simulink model "GHAME_Model_2018b"  (R2018b)
settings: Solver=ode2  StartTime=0.0  StopTime=Sim.simulation.duration  FixedStep=Sim.sample_time  RelTol=1e-3
undefined symbols (not defined in the file): Data, IC, Sim, UNC, v0_BE_B
libraries: simulink_extras x8, sharedutil x2
(part 1 of 2)
settings Model: PauseTimes=399.98  EnablePacing=on  PacingRate=5  Creator=Thoma  LastModifiedBy=muel_td
settings SolverCC: PositivePriorityOrder=on  MinimalZcImpactIntegration=on
settings DataIOCC: ExternalInput=getinputstruct(report2)  InitialState=getstatestruct(report2)  ReturnWorkspaceOutputs=on
settings OptimizationCC: SimCompilerOptimization=on  AccelVerboseBuild=on
settings DebuggingCC: RTPrefix=none  StringTruncationChecking=none  ReadBeforeWriteMsg=DisableAll  WriteAfterWriteMsg=DisableAll  WriteAfterReadMsg=DisableAll  AlgebraicLoopMsg=none  SignalResolutionControl=None  MultiTaskDSMMsg=none  IntegerOverflowMsg=none  ParameterDowncastMsg=none  ParameterOverflowMsg=none  ParameterPrecisionLossMsg=none  ParameterTunabilityLossMsg=none  UnconnectedInputMsg=none  UnconnectedOutputMsg=none  UnconnectedLineMsg=none  SFMachineParentedDataDiag=error  IntegerSaturationMsg=none
settings ModelReferenceCC: UpdateModelReferenceTargets=IfOutOfDate  EnableRefExpFcnMdlSchedulingChecks=off
settings SFSimCC: SFSimEcho=off
settings RTWCC: Description=Generic Real-Time Target

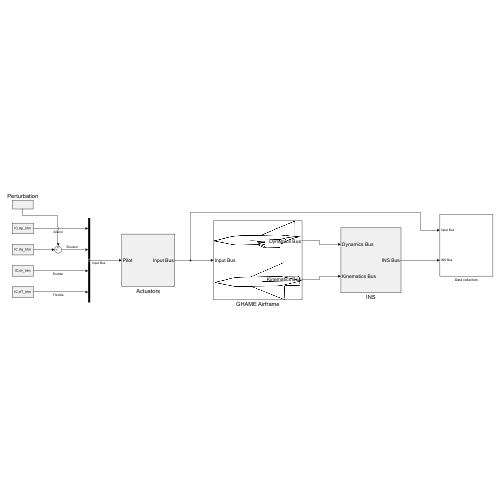
[thumbnail: Simulink's stored preview of the top-level diagram]
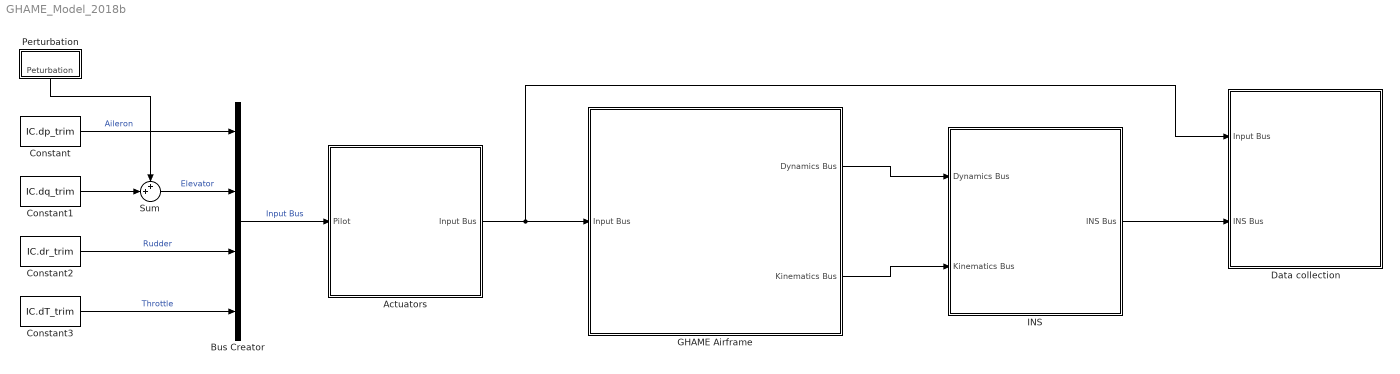
== system GHAME_Model_2018b ==
  Actuators : Subsystem
  Bus Creator : BusCreator  Inputs=4
  Constant : Constant  Value=IC.dp_trim  SampleTime=0
  Constant1 : Constant  Value=IC.dq_trim  SampleTime=0
  Constant2 : Constant  Value=IC.dr_trim  SampleTime=0
  Constant3 : Constant  Value=IC.dT_trim  SampleTime=0
  Data collection : Subsystem
  GHAME Airframe : Subsystem
      mask Display: image('GHAME.png'); % Use "Edit Image" on toolstrip to change.
  INS : Subsystem
  Perturbation : Subsystem
  Sum : Sum  Inputs=++|
  wires:
  Actuators/1(Input Bus) -> Data collection/1(Input Bus), GHAME Airframe/1(Input Bus)
  Constant/1 -> Bus Creator/1  "Aileron"
  Constant2/1 -> Bus Creator/3  "Rudder"
  Constant3/1 -> Bus Creator/4  "Throttle"
  Bus Creator/1 -> Actuators/1(Pilot)  "Input Bus"
  GHAME Airframe/2(Kinematics Bus) -> INS/2(Kinematics Bus)
  GHAME Airframe/1(Dynamics Bus) -> INS/1(Dynamics Bus)
  INS/1(INS Bus) -> Data collection/2(INS Bus)
  Constant1/1 -> Sum/2
  Perturbation/1(Peturbation) -> Sum/1
  Sum/1 -> Bus Creator/2  "Elevator"

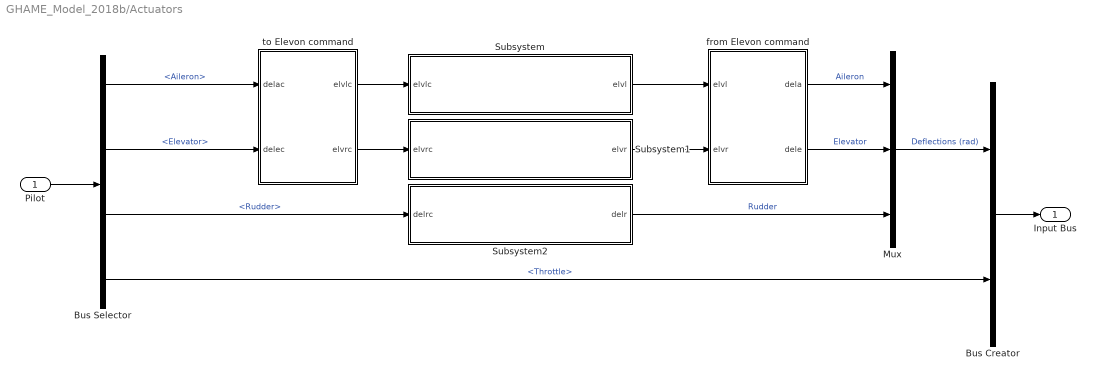
== system GHAME_Model_2018b/Actuators ==
  Pilot : Inport
  Bus Creator : BusCreator  Inputs=2
  Bus Selector : BusSelector  OutputSignals=Aileron,Elevator,Rudder,Throttle
  Mux : Mux  Inputs=3
  Subsystem : Subsystem
  Subsystem1 : Subsystem
  Subsystem2 : Subsystem
  from Elevon command : Subsystem
  to Elevon command : Subsystem
  Input Bus : Outport  PortDimensions=[4]
  wires:
  from Elevon command/1(dela) -> Mux/1  "Aileron"
  Bus Selector/3 -> Subsystem2/1(delrc)  "<Rudder>"
  to Elevon command/2(elvrc) -> Subsystem1/1(elvrc)
  Bus Selector/1 -> to Elevon command/1(delac)  "<Aileron>"
  to Elevon command/1(elvlc) -> Subsystem/1(elvlc)
  Bus Selector/2 -> to Elevon command/2(delec)  "<Elevator>"
  Subsystem/1(elvl) -> from Elevon command/1(elvl)
  Subsystem2/1(delr) -> Mux/3  "Rudder"
  Bus Creator/1 -> Input Bus/1
  Pilot/1 -> Bus Selector/1
  Bus Selector/4 -> Bus Creator/2  "<Throttle>"
  from Elevon command/2(dele) -> Mux/2  "Elevator"
  Subsystem1/1(elvr) -> from Elevon command/2(elvr)
  Mux/1 -> Bus Creator/1  "Deflections (rad)"

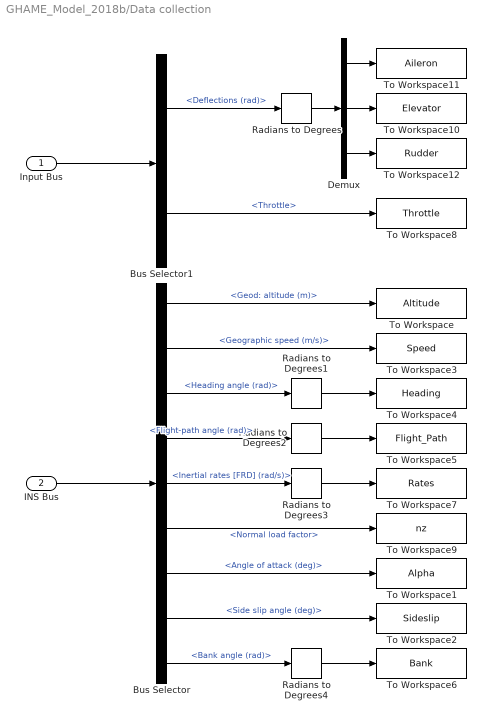
== system GHAME_Model_2018b/Data collection ==
  Input Bus : Inport
  INS Bus : Inport  Port=2
  Bus Selector : BusSelector  OutputSignals=Geod: altitude (m),Geographic speed (m/s),Heading angle (rad),Flight-path angle (rad),Inertial rates [FRD] (rad/s),Normal load factor,Angle of attack (deg),Side slip angle (deg),Bank angle (rad)
  Bus Selector1 : BusSelector  OutputSignals=Deflections (rad),Throttle
  Demux : Demux  Outputs=3
  Radians to Degrees{,1..4} (5 alike) : simulink_extras/Transformations/Radians to Degrees
  To Workspace : ToWorkspace  VariableName=Altitude  SampleTime=Sim.sample_time
  To Workspace1 : ToWorkspace  VariableName=Alpha  SampleTime=Sim.sample_time
  To Workspace10 : ToWorkspace  VariableName=Elevator  SampleTime=Sim.sample_time
  To Workspace11 : ToWorkspace  VariableName=Aileron  SampleTime=Sim.sample_time
  To Workspace12 : ToWorkspace  VariableName=Rudder  SampleTime=Sim.sample_time
  To Workspace2 : ToWorkspace  VariableName=Sideslip  SampleTime=Sim.sample_time
  To Workspace3 : ToWorkspace  VariableName=Speed  SampleTime=Sim.sample_time
  To Workspace4 : ToWorkspace  VariableName=Heading  SampleTime=Sim.sample_time
  To Workspace5 : ToWorkspace  VariableName=Flight_Path  SampleTime=Sim.sample_time
  To Workspace6 : ToWorkspace  VariableName=Bank  SampleTime=Sim.sample_time
  To Workspace7 : ToWorkspace  VariableName=Rates  SampleTime=Sim.sample_time
  To Workspace8 : ToWorkspace  VariableName=Throttle  SampleTime=Sim.sample_time
  To Workspace9 : ToWorkspace  VariableName=nz  SampleTime=Sim.sample_time
  wires:
  INS Bus/1 -> Bus Selector/1
  Bus Selector/1 -> To Workspace/1  "<Geod: altitude (m)>"
  Bus Selector/2 -> To Workspace3/1  "<Geographic speed (m/s)>"
  Bus Selector/3 -> Radians to Degrees1/1  "<Heading angle (rad)>"
  Bus Selector/4 -> Radians to Degrees2/1  "<Flight-path angle (rad)>"
  Bus Selector/5 -> Radians to Degrees3/1  "<Inertial rates [FRD] (rad/s)>"
  Bus Selector/6 -> To Workspace9/1  "<Normal load factor>"
  Bus Selector/7 -> To Workspace1/1  "<Angle of attack (deg)>"
  Bus Selector/8 -> To Workspace2/1  "<Side slip angle (deg)>"
  Bus Selector/9 -> Radians to Degrees4/1  "<Bank angle (rad)>"
  Input Bus/1 -> Bus Selector1/1
  Bus Selector1/1 -> Radians to Degrees/1  "<Deflections (rad)>"
  Demux/1 -> To Workspace11/1
  Demux/2 -> To Workspace10/1
  Demux/3 -> To Workspace12/1
  Radians to Degrees/1 -> Demux/1
  Bus Selector1/2 -> To Workspace8/1  "<Throttle>"
  Radians to Degrees1/1 -> To Workspace4/1
  Radians to Degrees2/1 -> To Workspace5/1
  Radians to Degrees3/1 -> To Workspace7/1
  Radians to Degrees4/1 -> To Workspace6/1

== system GHAME_Model_2018b/GHAME Airframe ==
  Input Bus : Inport
  Dynamics : Subsystem  Priority=4
  Environment : Subsystem  Priority=1
  Forces and Moments : Subsystem
  Kinematics : Subsystem  Priority=2
  Dynamics Bus : Outport
  Kinematics Bus : Outport  Port=2
  wires:
  Kinematics/1(Kinematics Bus) -> Forces and Moments/4(Kinematics Bus), Environment/2(Kinematics Bus), Kinematics Bus/1, Dynamics/3(Kinematics Bus)
  Dynamics/1(Dynamics Bus) -> Dynamics Bus/1, Forces and Moments/2(Dynamics Bus), Environment/1(Dynamics Bus), Kinematics/2(Dynamics Bus)
  Environment/1(Environment Bus) -> Forces and Moments/3(Environment Bus), Dynamics/2(Environment Bus), Kinematics/1(Environment Bus)
  Forces and Moments/1(Force Bus) -> Dynamics/1(Force Bus)
  Input Bus/1 -> Forces and Moments/1(Input Bus)

== system GHAME_Model_2018b/INS ==
  Dynamics Bus : Inport
  Kinematics Bus : Inport  Port=2
  Bus Creator : BusCreator  Inputs=12
  Bus Selector : BusSelector  OutputSignals=Newton Bus.Inertial position (m),Euler Bus.Vehicle angular vel: wrt Inertial [FRD] (rad/s),Newton Bus.Inertial velocity (m/s),Newton Bus.Specific Force [FRD]
  Bus Selector1 : BusSelector  OutputSignals=TM of body wrt inertial coord:
  INS : Subsystem
  INS Bus : Outport
  wires:
  INS/4(FSPCB) -> Bus Creator/4  "Specific force [FRD]"
  INS/5(thtvdc) -> Bus Creator/5  "Flight-path angle (rad)"
  INS/2(dvbec) -> Bus Creator/2  "Geographic speed (m/s)"
  INS/3(alphacx) -> Bus Creator/3  "Angle of attack (deg)"
  INS/1(WBICB) -> Bus Creator/1  "Inertial rates [FRD] (rad/s)"
  INS/7(psivdc) -> Bus Creator/7  "Heading angle (rad)"
  INS/6(betacx) -> Bus Creator/6  "Side slip angle (deg)"
  INS/11(muc) -> Bus Creator/11  "Bank angle (rad)"
  INS/9(lonc) -> Bus Creator/9  "Longitude (rad)"
  INS/8(altc) -> Bus Creator/8  "Geod: altitude (m)"
  INS/10(latc) -> Bus Creator/10  "Geod: latitude (rad)"
  Bus Selector/1 -> INS/2(SBII)  "<Inertial position (m)>"
  Bus Selector/3 -> INS/4(VBII)  "<Inertial velocity (m/s)>"
  Dynamics Bus/1 -> Bus Selector/1
  Bus Selector/2 -> INS/3(WBIB)  "<Vehicle angular vel: wrt Inertial [FRD] (rad/s)>"
  Bus Selector/4 -> INS/5(FSPB)  "<Specific Force [FRD]>"
  Kinematics Bus/1 -> Bus Selector1/1
  Bus Selector1/1 -> INS/1(TBI)  "<TM of body wrt inertial coord:>"
  Bus Creator/1 -> INS Bus/1
  INS/12(nzc) -> Bus Creator/12  "Normal load factor"

== system GHAME_Model_2018b/Perturbation ==
  From Workspace : FromWorkspace  VariableName=CMD.perturbElevator.time_signal  SampleTime=Sim.sample_time
  Peturbation : Outport
  wires:
  From Workspace/1 -> Peturbation/1

== system GHAME_Model_2018b/Actuators/Subsystem ==
  elvlc : Inport
  2*zeta * wn : Gain  Gain=2*Sim.actuator.zeta*Sim.actuator.omega  SaturateOnIntegerOverflow=on  OutDataTypeStr=Inherit: Same as input  ParamDataTypeStr=Inherit: Same as input
  Demand limits : Saturate  UpperLimit=Sim.actuator.deflection_limit_deg*Sim.constants.RAD  LowerLimit=-Sim.actuator.deflection_limit_deg*Sim.constants.RAD
  "Integrator, Second-Order Limited" : SecondOrderIntegrator  ICX=IC.dp_trim+IC.dq_trim  LimitX=on  UpperLimitX=Sim.actuator.deflection_limit_deg*Sim.constants.RAD  LowerLimitX=-Sim.actuator.deflection_limit_deg*Sim.constants.RAD  ICDXDT=0  LimitDXDT=on  UpperLimitDXDT=Sim.actuator.deflection_rate_limit_deg*Sim.constants.RAD  LowerLimitDXDT=-Sim.actuator.deflection_rate_limit_deg*Sim.constants.RAD
  Sum2 : Sum  Inputs=|+-  InputSameDT=on  SaturateOnIntegerOverflow=on  OutDataTypeStr=Inherit: Same as first input
  Sum3 : Sum  Inputs=|+-  InputSameDT=on  SaturateOnIntegerOverflow=on  OutDataTypeStr=Inherit: Same as first input
  rate limit*2*zeta/wn : Saturate  UpperLimit=Sim.actuator.deflection_rate_limit_deg*2*Sim.actuator.zeta/Sim.actuator.omega*Sim.constants.RAD  LowerLimit=-Sim.actuator.deflection_rate_limit_deg*2*Sim.actuator.zeta/Sim.actuator.omega*Sim.constants.RAD
  wn^2 : Gain  Gain=Sim.actuator.omega^2  SaturateOnIntegerOverflow=on  OutDataTypeStr=Inherit: Same as input  ParamDataTypeStr=Inherit: Same as input
  elvl : Outport
  wires:
  wn^2/1 -> Sum2/1
  Sum3/1 -> rate limit*2*zeta/wn/1
  Sum2/1 -> "Integrator, Second-Order Limited"/1
  Demand limits/1 -> Sum3/1
  "Integrator, Second-Order Limited"/2 -> 2*zeta * wn/1
  "Integrator, Second-Order Limited"/1 -> Sum3/2, elvl/1
  2*zeta * wn/1 -> Sum2/2
  rate limit*2*zeta/wn/1 -> wn^2/1
  elvlc/1 -> Demand limits/1

== system GHAME_Model_2018b/Actuators/Subsystem1 ==
  elvrc : Inport
  2*zeta * wn : Gain  Gain=2*Sim.actuator.zeta*Sim.actuator.omega  SaturateOnIntegerOverflow=on  OutDataTypeStr=Inherit: Same as input  ParamDataTypeStr=Inherit: Same as input
  Demand limits : Saturate  UpperLimit=Sim.actuator.deflection_limit_deg*Sim.constants.RAD  LowerLimit=-Sim.actuator.deflection_limit_deg*Sim.constants.RAD
  "Integrator, Second-Order Limited" : SecondOrderIntegrator  ICX=IC.dq_trim-IC.dp_trim  LimitX=on  UpperLimitX=Sim.actuator.deflection_limit_deg*Sim.constants.RAD  LowerLimitX=-Sim.actuator.deflection_limit_deg*Sim.constants.RAD  ICDXDT=0  LimitDXDT=on  UpperLimitDXDT=Sim.actuator.deflection_rate_limit_deg*Sim.constants.RAD  LowerLimitDXDT=-Sim.actuator.deflection_rate_limit_deg*Sim.constants.RAD
  Sum2 : Sum  Inputs=|+-  InputSameDT=on  SaturateOnIntegerOverflow=on  OutDataTypeStr=Inherit: Same as first input
  Sum3 : Sum  Inputs=|+-  InputSameDT=on  SaturateOnIntegerOverflow=on  OutDataTypeStr=Inherit: Same as first input
  rate limit*2*zeta/wn : Saturate  UpperLimit=Sim.actuator.deflection_rate_limit_deg*2*Sim.actuator.zeta/Sim.actuator.omega*Sim.constants.RAD  LowerLimit=-Sim.actuator.deflection_rate_limit_deg*2*Sim.actuator.zeta/Sim.actuator.omega*Sim.constants.RAD
  wn^2 : Gain  Gain=Sim.actuator.omega^2  SaturateOnIntegerOverflow=on  OutDataTypeStr=Inherit: Same as input  ParamDataTypeStr=Inherit: Same as input
  elvr : Outport
  wires:
  2*zeta * wn/1 -> Sum2/2
  rate limit*2*zeta/wn/1 -> wn^2/1
  "Integrator, Second-Order Limited"/2 -> 2*zeta * wn/1
  wn^2/1 -> Sum2/1
  "Integrator, Second-Order Limited"/1 -> elvr/1, Sum3/2
  Demand limits/1 -> Sum3/1
  elvrc/1 -> Demand limits/1
  Sum2/1 -> "Integrator, Second-Order Limited"/1
  Sum3/1 -> rate limit*2*zeta/wn/1

== system GHAME_Model_2018b/Actuators/Subsystem2 ==
  delrc : Inport
  2*zeta * wn : Gain  Gain=2*Sim.actuator.zeta*Sim.actuator.omega  SaturateOnIntegerOverflow=on  OutDataTypeStr=Inherit: Same as input  ParamDataTypeStr=Inherit: Same as input
  Demand limits : Saturate  UpperLimit=Sim.actuator.deflection_limit_deg*Sim.constants.RAD  LowerLimit=-Sim.actuator.deflection_limit_deg*Sim.constants.RAD
  "Integrator, Second-Order Limited" : SecondOrderIntegrator  ICX=IC.dr_trim  LimitX=on  UpperLimitX=Sim.actuator.deflection_limit_deg*Sim.constants.RAD  LowerLimitX=-Sim.actuator.deflection_limit_deg*Sim.constants.RAD  ICDXDT=0  LimitDXDT=on  UpperLimitDXDT=Sim.actuator.deflection_rate_limit_deg*Sim.constants.RAD  LowerLimitDXDT=-Sim.actuator.deflection_rate_limit_deg*Sim.constants.RAD
  Sum2 : Sum  Inputs=|+-  InputSameDT=on  SaturateOnIntegerOverflow=on  OutDataTypeStr=Inherit: Same as first input
  Sum3 : Sum  Inputs=|+-  InputSameDT=on  SaturateOnIntegerOverflow=on  OutDataTypeStr=Inherit: Same as first input
  rate limit*2*zeta/wn : Saturate  UpperLimit=Sim.actuator.deflection_rate_limit_deg*2*Sim.actuator.zeta/Sim.actuator.omega*Sim.constants.RAD  LowerLimit=-Sim.actuator.deflection_rate_limit_deg*2*Sim.actuator.zeta/Sim.actuator.omega*Sim.constants.RAD
  wn^2 : Gain  Gain=Sim.actuator.omega^2  SaturateOnIntegerOverflow=on  OutDataTypeStr=Inherit: Same as input  ParamDataTypeStr=Inherit: Same as input
  delr : Outport
  wires:
  delrc/1 -> Demand limits/1
  Sum2/1 -> "Integrator, Second-Order Limited"/1
  Sum3/1 -> rate limit*2*zeta/wn/1
  "Integrator, Second-Order Limited"/2 -> 2*zeta * wn/1
  rate limit*2*zeta/wn/1 -> wn^2/1
  2*zeta * wn/1 -> Sum2/2
  wn^2/1 -> Sum2/1
  "Integrator, Second-Order Limited"/1 -> delr/1, Sum3/2
  Demand limits/1 -> Sum3/1

== system GHAME_Model_2018b/Actuators/from Elevon command ==
  elvl : Inport
  elvr : Inport  Port=2
  Add : Sum  Inputs=+-
  Add1 : Sum
  Constant : Constant  Value=2
  Divide : Product  Inputs=*/
  Divide1 : Product  Inputs=/*
  dela : Outport
  dele : Outport  Port=2
  wires:
  Add/1 -> Divide/1
  Add1/1 -> Divide1/2
  elvl/1 -> Add/1, Add1/2
  elvr/1 -> Add/2, Add1/1
  Divide/1 -> dela/1
  Constant/1 -> Divide1/1, Divide/2
  Divide1/1 -> dele/1

== system GHAME_Model_2018b/Actuators/to Elevon command ==
  delac : Inport
  delec : Inport  Port=2
  Add : Sum
  Add1 : Sum
  Unary Minus : UnaryMinus
  elvlc : Outport
  elvrc : Outport  Port=2
  wires:
  Add1/1 -> elvrc/1
  delac/1 -> Unary Minus/1, Add/1
  Unary Minus/1 -> Add1/2
  delec/1 -> Add1/1, Add/2
  Add/1 -> elvlc/1

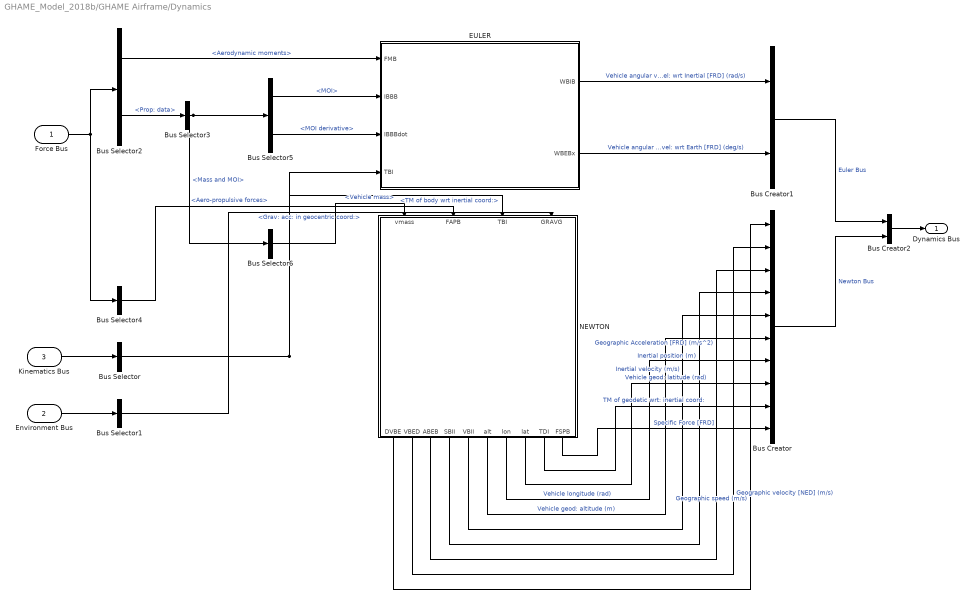
== system GHAME_Model_2018b/GHAME Airframe/Dynamics ==
  Force Bus : Inport
  Environment Bus : Inport  Port=2
  Kinematics Bus : Inport  Port=3
  Bus Creator : BusCreator  Inputs=10
  Bus Creator1 : BusCreator  Inputs=2
  Bus Creator2 : BusCreator  Inputs=2
  Bus Selector : BusSelector  OutputSignals=TM of body wrt inertial coord:
  Bus Selector1 : BusSelector  OutputSignals=Grav: acc: in geocentric coord:
  Bus Selector2 : BusSelector  OutputSignals=Aerodynamic moments,Prop: data
  Bus Selector3 : BusSelector  OutputSignals=Mass and MOI
  Bus Selector4 : BusSelector  OutputSignals=Aero-propulsive forces
  Bus Selector5 : BusSelector  OutputSignals=MOI,MOI derivative
  Bus Selector6 : BusSelector  OutputSignals=Vehicle mass
  EULER : Subsystem
  NEWTON : Subsystem
  Dynamics Bus : Outport
  wires:
  Bus Creator/1 -> Bus Creator2/2  "Newton Bus"
  EULER/2(WBEBx) -> Bus Creator1/2  "Vehicle angular vel: wrt Earth [FRD] (deg/s)"
  Kinematics Bus/1 -> Bus Selector/1
  Bus Selector/1 -> NEWTON/3(TBI), EULER/4(TBI)  "<TM of body wrt inertial coord:>"
  Bus Selector1/1 -> NEWTON/4(GRAVG)  "<Grav: acc: in geocentric coord:>"
  EULER/1("WBIB ") -> Bus Creator1/1  "Vehicle angular vel: wrt Inertial [FRD] (rad/s)"
  Environment Bus/1 -> Bus Selector1/1
  Bus Creator1/1 -> Bus Creator2/1  "Euler Bus"
  Bus Creator2/1 -> Dynamics Bus/1
  NEWTON/4("SBII ") -> Bus Creator/4  "Inertial position (m)"
  NEWTON/7(lon) -> Bus Creator/7  "Vehicle longitude (rad)"
  NEWTON/8(lat) -> Bus Creator/8  "Vehicle geod: latitude (rad)"
  NEWTON/6(alt) -> Bus Creator/6  "Vehicle geod: altitude (m)"
  NEWTON/9(TDI) -> Bus Creator/9  "TM of geodetic wrt: inertial coord:"
  NEWTON/2(VBED) -> Bus Creator/2  "Geographic velocity [NED] (m/s)"
  NEWTON/3(ABEB) -> Bus Creator/3  "Geographic Acceleration [FRD] (m/s^2)"
  NEWTON/1(DVBE) -> Bus Creator/1  "Geographic speed (m/s)"
  Force Bus/1 -> Bus Selector2/1, Bus Selector4/1
  Bus Selector2/1 -> EULER/1(FMB)  "<Aerodynamic moments>"
  Bus Selector2/2 -> Bus Selector3/1  "<Prop: data>"
  Bus Selector4/1 -> NEWTON/2(FAPB)  "<Aero-propulsive forces>"
  NEWTON/10(FSPB) -> Bus Creator/10  "Specific Force [FRD]"
  NEWTON/5(VBII) -> Bus Creator/5  "Inertial velocity (m/s)"
  Bus Selector3/1 -> Bus Selector5/1, Bus Selector6/1  "<Mass and MOI>"
  Bus Selector5/1 -> EULER/2(IBBB)  "<MOI>"
  Bus Selector5/2 -> EULER/3(IBBBdot)  "<MOI derivative>"
  Bus Selector6/1 -> NEWTON/1(vmass)  "<Vehicle mass>"

== system GHAME_Model_2018b/GHAME Airframe/Environment ==
  Dynamics Bus : Inport
  Kinematics Bus : Inport  Port=2
  Bus Creator : BusCreator  Inputs=6
  Bus Selector : BusSelector  OutputSignals=Newton Bus.Inertial position (m),Newton Bus.Vehicle geod: altitude (m),Newton Bus.Vehicle geod: latitude (rad),Newton Bus.Vehicle longitude (rad),Newton Bus.Geographic velocity [NED] (m/s)
  Bus Selector1 : BusSelector  OutputSignals=Total angle of attack (deg),TM of body wrt geodetic coord:,Aeroballistic roll angle (deg)
  ENVIRONMENT : Subsystem  Priority=1
  Environment Bus : Outport
  wires:
  Dynamics Bus/1 -> Bus Selector/1
  Bus Creator/1 -> Environment Bus/1
  ENVIRONMENT/1(GRAVG) -> Bus Creator/1  "Grav: acc: in geocentric coord:"
  ENVIRONMENT/2(rho) -> Bus Creator/2  "Atmospheric density"
  ENVIRONMENT/3(pdynmc) -> Bus Creator/3  "Dynamic pressure"
  ENVIRONMENT/4(vmach) -> Bus Creator/4  "Mach number"
  ENVIRONMENT/5(DVBA) -> Bus Creator/5  "Speed of vehicle wrt air"
  Bus Selector/1 -> ENVIRONMENT/1(SBII)  "<Inertial position (m)>"
  Bus Selector/2 -> ENVIRONMENT/2(alt)  "<Vehicle geod: altitude (m)>"
  Bus Selector/5 -> ENVIRONMENT/5(VBED)  "<Geographic velocity [NED] (m/s)>"
  Bus Selector/4 -> ENVIRONMENT/4(lon)  "<Vehicle longitude (rad)>"
  Bus Selector/3 -> ENVIRONMENT/3(lat)  "<Vehicle geod: latitude (rad)>"
  Kinematics Bus/1 -> Bus Selector1/1
  Bus Selector1/2 -> ENVIRONMENT/7(TBD)  "<TM of body wrt geodetic coord:>"
  Bus Selector1/3 -> ENVIRONMENT/8(phipx)  "<Aeroballistic roll angle (deg)>"
  Bus Selector1/1 -> ENVIRONMENT/6(alppx)  "<Total angle of attack (deg)>"
  ENVIRONMENT/6(VBAB) -> Bus Creator/6  "Velocity of veh: wrt air [FRD]"

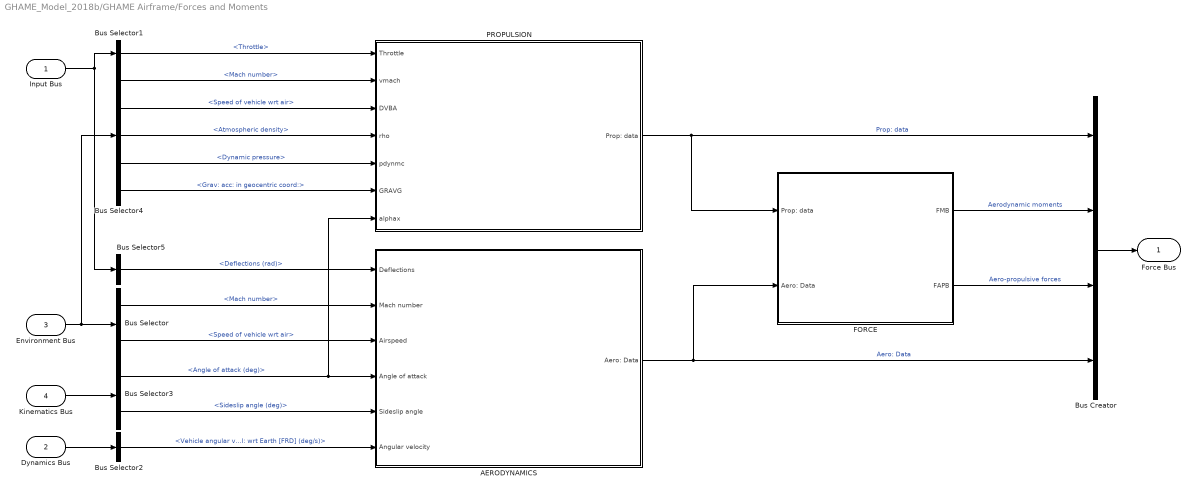
== system GHAME_Model_2018b/GHAME Airframe/Forces and Moments ==
  Input Bus : Inport
  Dynamics Bus : Inport  Port=2
  Environment Bus : Inport  Port=3
  Kinematics Bus : Inport  Port=4
  AERODYNAMICS : Subsystem
  Bus Creator : BusCreator  Inputs=4
  Bus Selector : BusSelector  OutputSignals=Mach number,Speed of vehicle wrt air
  Bus Selector1 : BusSelector  OutputSignals=Throttle
  Bus Selector2 : BusSelector  OutputSignals=Euler Bus.Vehicle angular vel: wrt Earth [FRD] (deg/s)
  Bus Selector3 : BusSelector  OutputSignals=Angle of attack (deg),Sideslip angle (deg)
  Bus Selector4 : BusSelector  OutputSignals=Mach number,Speed of vehicle wrt air,Atmospheric density,Dynamic pressure,Grav: acc: in geocentric coord:
  Bus Selector5 : BusSelector  OutputSignals=Deflections (rad)
  FORCE : Subsystem
  PROPULSION : Subsystem
  Force Bus : Outport
  wires:
  FORCE/2(FAPB) -> Bus Creator/3  "Aero-propulsive forces"
  Environment Bus/1 -> Bus Selector4/1, Bus Selector/1
  Bus Selector/2 -> AERODYNAMICS/3(Airspeed)  "<Speed of vehicle wrt air>"
  Dynamics Bus/1 -> Bus Selector2/1
  Kinematics Bus/1 -> Bus Selector3/1
  Input Bus/1 -> Bus Selector1/1, Bus Selector5/1
  Bus Selector3/1 -> PROPULSION/7(alphax), AERODYNAMICS/4(Angle of attack)  "<Angle of attack (deg)>"
  Bus Selector4/4 -> PROPULSION/5(pdynmc)  "<Dynamic pressure>"
  FORCE/1(FMB) -> Bus Creator/2  "Aerodynamic moments"
  PROPULSION/1(Prop: data) -> FORCE/1(Prop: data), Bus Creator/1  "Prop: data"
  AERODYNAMICS/1(Aero: Data) -> Bus Creator/4, FORCE/2(Aero: Data)  "Aero: Data"
  Bus Creator/1 -> Force Bus/1
  Bus Selector1/1 -> PROPULSION/1(Throttle)  "<Throttle>"
  Bus Selector/1 -> AERODYNAMICS/2(Mach number)  "<Mach number>"
  Bus Selector4/3 -> PROPULSION/4(rho)  "<Atmospheric density>"
  Bus Selector3/2 -> AERODYNAMICS/5(Sideslip angle)  "<Sideslip angle (deg)>"
  Bus Selector2/1 -> AERODYNAMICS/6(Angular velocity)  "<Vehicle angular vel: wrt Earth [FRD] (deg/s)>"
  Bus Selector4/2 -> PROPULSION/3(DVBA)  "<Speed of vehicle wrt air>"
  Bus Selector4/1 -> PROPULSION/2(vmach)  "<Mach number>"
  Bus Selector4/5 -> PROPULSION/6(GRAVG)  "<Grav: acc: in geocentric coord:>"
  Bus Selector5/1 -> AERODYNAMICS/1(Deflections)  "<Deflections (rad)>"

== system GHAME_Model_2018b/GHAME Airframe/Kinematics ==
  Environment Bus : Inport
  Dynamics Bus : Inport  Port=2
  Bus Creator : BusCreator  Inputs=7
  Bus Selector : BusSelector  OutputSignals=Velocity of veh: wrt air [FRD]
  Bus Selector1 : BusSelector  OutputSignals=Newton Bus.Vehicle longitude (rad),Newton Bus.Vehicle geod: latitude (rad),Euler Bus.Vehicle angular vel: wrt Inertial [FRD] (rad/s)
  KINEMATICS : Subsystem
  Kinematics Bus : Outport
  wires:
  Bus Creator/1 -> Kinematics Bus/1
  Environment Bus/1 -> Bus Selector/1
  Dynamics Bus/1 -> Bus Selector1/1
  Bus Selector/1 -> KINEMATICS/1(VBAB)  "<Velocity of veh: wrt air [FRD]>"
  KINEMATICS/3(alphax) -> Bus Creator/3  "Angle of attack (deg)"
  KINEMATICS/1("TBI ") -> Bus Creator/1  "TM of body wrt inertial coord:"
  KINEMATICS/2(TBD) -> Bus Creator/2  "TM of body wrt geodetic coord:"
  KINEMATICS/5(alppx) -> Bus Creator/5  "Total angle of attack (deg)"
  KINEMATICS/6(phipx) -> Bus Creator/6  "Aeroballistic roll angle (deg)"
  KINEMATICS/4(betax) -> Bus Creator/4  "Sideslip angle (deg)"
  Bus Selector1/1 -> KINEMATICS/2(lon)  "<Vehicle longitude (rad)>"
  Bus Selector1/2 -> KINEMATICS/3(lat)  "<Vehicle geod: latitude (rad)>"
  Bus Selector1/3 -> KINEMATICS/4(WBIB)  "<Vehicle angular vel: wrt Inertial [FRD] (rad/s)>"
  KINEMATICS/7(phibdx) -> Bus Creator/7  "Body roll angle (deg)"

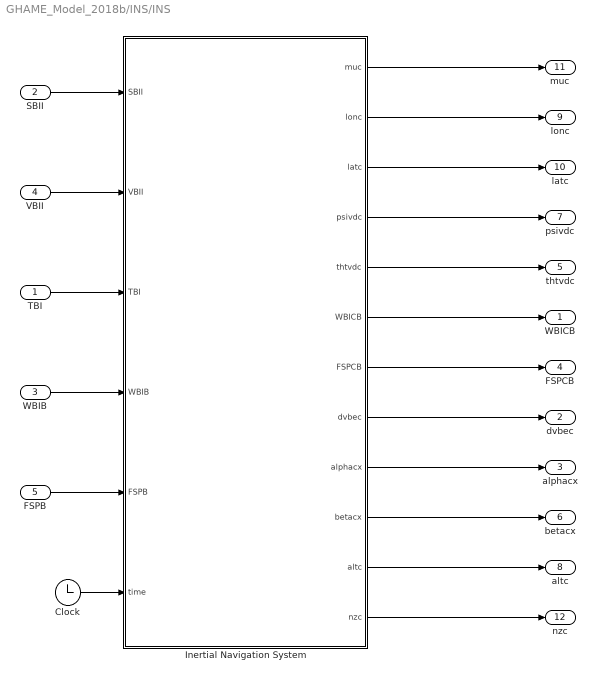
== system GHAME_Model_2018b/INS/INS ==
  TBI : Inport
  SBII : Inport  Port=2
  WBIB : Inport  Port=3
  VBII : Inport  Port=4
  FSPB : Inport  Port=5
  Clock : Clock
  Inertial Navigation System : MATLAB Function  TreatAsAtomicUnit=on
  WBICB : Outport
  dvbec : Outport  Port=2
  alphacx : Outport  Port=3
  FSPCB : Outport  Port=4
  thtvdc : Outport  Port=5
  betacx : Outport  Port=6
  psivdc : Outport  Port=7
  altc : Outport  Port=8
  lonc : Outport  Port=9
  latc : Outport  Port=10
  muc : Outport  Port=11
  nzc : Outport  Port=12
  wires:
  SBII/1 -> Inertial Navigation System/1(SBII)
  VBII/1 -> Inertial Navigation System/2(VBII)
  TBI/1 -> Inertial Navigation System/3(TBI)
  Clock/1 -> Inertial Navigation System/6(time)
  WBIB/1 -> Inertial Navigation System/4(WBIB)
  FSPB/1 -> Inertial Navigation System/5(FSPB)
  Inertial Navigation System/2(lonc) -> lonc/1
  Inertial Navigation System/12(nzc) -> nzc/1
  Inertial Navigation System/11(altc) -> altc/1
  Inertial Navigation System/10(betacx) -> betacx/1
  Inertial Navigation System/9(alphacx) -> alphacx/1
  Inertial Navigation System/8(dvbec) -> dvbec/1
  Inertial Navigation System/7(FSPCB) -> FSPCB/1
  Inertial Navigation System/6(WBICB) -> WBICB/1
  Inertial Navigation System/1(muc) -> muc/1
  Inertial Navigation System/3(latc) -> latc/1
  Inertial Navigation System/4(psivdc) -> psivdc/1
  Inertial Navigation System/5(thtvdc) -> thtvdc/1

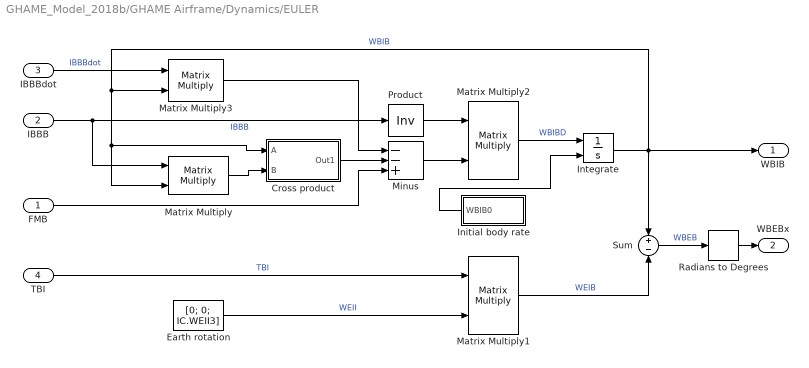
== system GHAME_Model_2018b/GHAME Airframe/Dynamics/EULER ==
  FMB : Inport
  IBBB : Inport  Port=2
  IBBBdot : Inport  Port=3
  TBI : Inport  Port=4
  Cross product : Subsystem
  Earth rotation : Constant  Value=[0; 0; IC.WEII3]
  Initial body rate : Subsystem
  Integrate : Integrator  InitialConditionSource=external  InitialCondition=v0_BE_B
  Matrix Multiply{,1..3} (4 alike) : Product  Multiplication=Matrix(*)
  Minus : Sum  Inputs=--+
  Product : Product  Inputs=/  Multiplication=Matrix(*)  SaturateOnIntegerOverflow=on  OutDataTypeStr=Inherit: Same as first input
  Radians to Degrees : simulink_extras/Transformations/Radians to Degrees
  Sum : Sum  Inputs=+-
  "WBIB " : Outport
  WBEBx : Outport  Port=2
  wires:
  TBI/1 -> Matrix Multiply1/1  "TBI"
  Matrix Multiply1/1 -> Sum/2  "WEIB"
  FMB/1 -> Minus/3
  Matrix Multiply2/1 -> Integrate/1  "WBIBD"
  IBBB/1 -> Product/1, Matrix Multiply/1  "IBBB"
  Integrate/1 -> Sum/1, "WBIB "/1, Matrix Multiply3/2, Cross product/1(A), Matrix Multiply/2  "WBIB"
  Earth rotation/1 -> Matrix Multiply1/2  "WEII"
  Product/1 -> Matrix Multiply2/1
  Matrix Multiply/1 -> Cross product/2(B)
  Cross product/1(Out1) -> Minus/2
  Minus/1 -> Matrix Multiply2/2
  Radians to Degrees/1 -> WBEBx/1
  Sum/1 -> Radians to Degrees/1  "WBEB"
  IBBBdot/1 -> Matrix Multiply3/1  "IBBBdot"
  Matrix Multiply3/1 -> Minus/1
  Initial body rate/1(WBIB0) -> Integrate/2

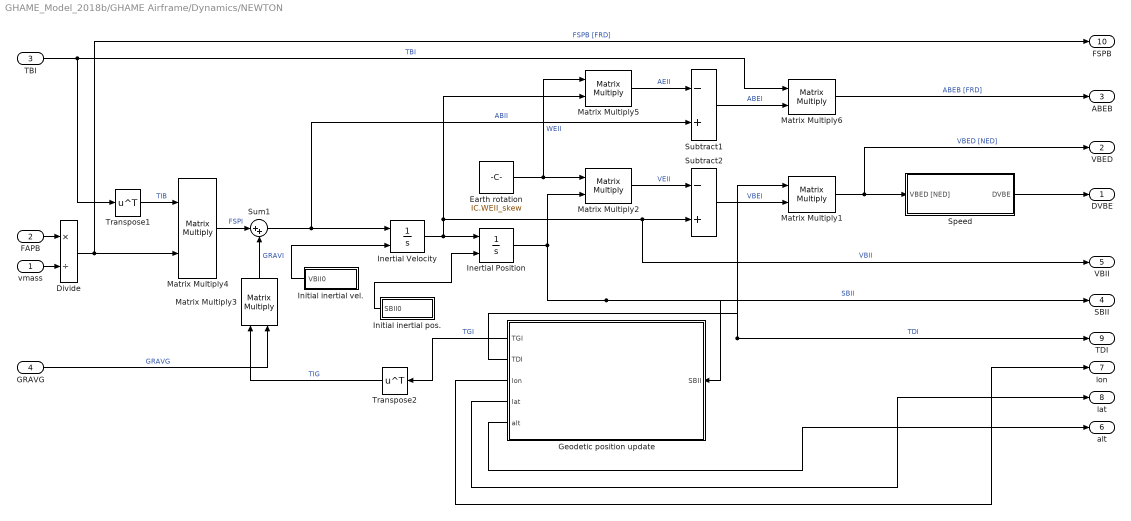
== system GHAME_Model_2018b/GHAME Airframe/Dynamics/NEWTON ==
  vmass : Inport
  FAPB : Inport  Port=2
  TBI : Inport  Port=3
  GRAVG : Inport  Port=4
  Divide : Product  Inputs=*/
  Earth rotation : Constant  Value=IC.WEII_skew
  Geodetic position update : Subsystem
  Inertial Position : Integrator  InitialConditionSource=external  InitialCondition=IC.SBII
  Inertial Velocity : Integrator  InitialConditionSource=external  InitialCondition=v0_BE_B
  Initial inertial pos. : Subsystem
  Initial inertial vel. : Subsystem
  Matrix Multiply{1..6} (6 alike) : Product  Multiplication=Matrix(*)
  Speed : Subsystem
  Subtract1 : Sum  Inputs=-+
  Subtract2 : Sum  Inputs=-+
  Sum1 : Sum  Inputs=|++
  Transpose1 : Math  Operator=transpose  SaturateOnIntegerOverflow=on
  Transpose2 : Math  Operator=transpose  SaturateOnIntegerOverflow=on
  DVBE : Outport
  VBED : Outport  Port=2
  ABEB : Outport  Port=3
  "SBII " : Outport  Port=4
  VBII : Outport  Port=5
  alt : Outport  Port=6
  lon : Outport  Port=7
  lat : Outport  Port=8
  TDI : Outport  Port=9
  FSPB : Outport  Port=10
  wires:
  Subtract2/1 -> Matrix Multiply1/2  "VBEI"
  Transpose1/1 -> Matrix Multiply4/1  "TIB"
  Inertial Position/1 -> Matrix Multiply2/2, Geodetic position update/1(SBII), "SBII "/1  "SBII"
  GRAVG/1 -> Matrix Multiply3/2  "GRAVG"
  Divide/1 -> Matrix Multiply4/2, FSPB/1  "FSPB [FRD]"
  Matrix Multiply4/1 -> Sum1/1  "FSPI"
  vmass/1 -> Divide/2
  Matrix Multiply2/1 -> Subtract2/1  "VEII"
  Matrix Multiply1/1 -> VBED/1, Speed/1(VBED [NED])  "VBED [NED]"
  FAPB/1 -> Divide/1
  Matrix Multiply3/1 -> Sum1/2  "GRAVI"
  Transpose2/1 -> Matrix Multiply3/1  "TIG"
  Geodetic position update/1(TGI) -> Transpose2/1  "TGI"
  Geodetic position update/5(alt) -> alt/1
  Geodetic position update/4(lat) -> lat/1
  Geodetic position update/3(lon) -> lon/1
  Geodetic position update/2(TDI) -> TDI/1, Matrix Multiply1/1  "TDI"
  Inertial Velocity/1 -> Inertial Position/1, Matrix Multiply5/2, Subtract2/2, VBII/1  "VBII"
  Sum1/1 -> Subtract1/2, Inertial Velocity/1  "ABII"
  Subtract1/1 -> Matrix Multiply6/2  "ABEI"
  Matrix Multiply5/1 -> Subtract1/1  "AEII"
  Earth rotation/1 -> Matrix Multiply5/1, Matrix Multiply2/1  "WEII"
  TBI/1 -> Matrix Multiply6/1, Transpose1/1  "TBI"
  Matrix Multiply6/1 -> ABEB/1  "ABEB [FRD]"
  Initial inertial vel./1(VBII0) -> Inertial Velocity/2
  Initial inertial pos./1(SBII0) -> Inertial Position/2
  Speed/1(DVBE) -> DVBE/1

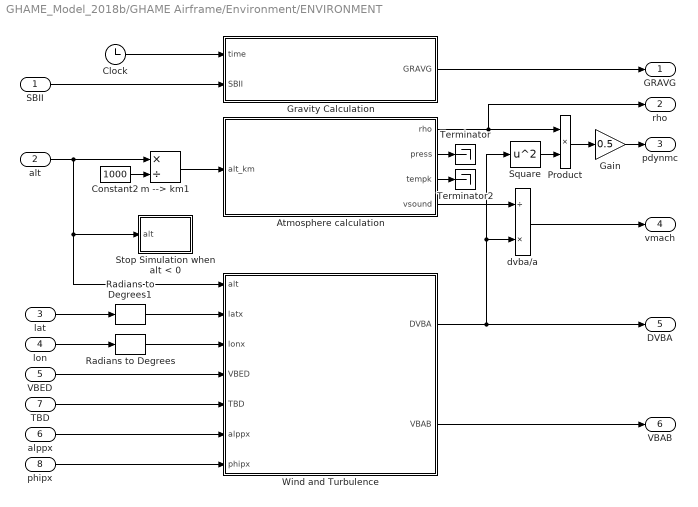
== system GHAME_Model_2018b/GHAME Airframe/Environment/ENVIRONMENT ==
  SBII : Inport
  alt : Inport  Port=2
  lat : Inport  Port=3
  lon : Inport  Port=4
  VBED : Inport  Port=5
  alppx : Inport  Port=6
  TBD : Inport  Port=7
  phipx : Inport  Port=8
  Atmosphere calculation : MATLAB Function  Priority=2  TreatAsAtomicUnit=on
  Clock : Clock
      settings: Priority=1
  Constant2 : Constant  Value=1000
  Gain : Gain  Gain=0.5
  Gravity Calculation : MATLAB Function  Priority=1  TreatAsAtomicUnit=on
  Product : Product
  Radians to Degrees : simulink_extras/Transformations/Radians to Degrees
  Radians to Degrees1 : simulink_extras/Transformations/Radians to Degrees
  Square : Math  Operator=square  SaturateOnIntegerOverflow=on
  Stop Simulation when alt < 0 : Subsystem
  Terminator : Terminator
  Terminator2 : Terminator
  Wind and Turbulence : Subsystem
  dvba/a : Product  Inputs=/*
  m --> km1 : Product  Inputs=*/
  GRAVG : Outport
  rho : Outport  Port=2
  pdynmc : Outport  Port=3
  vmach : Outport  Port=4
  DVBA : Outport  Port=5
  VBAB : Outport  Port=6
  wires:
  Clock/1 -> Gravity Calculation/1(time)
  SBII/1 -> Gravity Calculation/2(SBII)
  Constant2/1 -> m --> km1/2
  m --> km1/1 -> Atmosphere calculation/1(alt_km)
  Atmosphere calculation/4(vsound) -> dvba/a/1
  dvba/a/1 -> vmach/1
  Atmosphere calculation/1(rho) -> Product/1, rho/1
  Gravity Calculation/1(GRAVG) -> GRAVG/1
  Atmosphere calculation/3(tempk) -> Terminator2/1
  Atmosphere calculation/2(press) -> Terminator/1
  alt/1 -> Wind and Turbulence/1(alt), Stop Simulation when alt < 0/1(alt), m --> km1/1
  Wind and Turbulence/1(DVBA) -> DVBA/1, dvba/a/2, Square/1
  VBED/1 -> Wind and Turbulence/4(VBED)
  lat/1 -> Radians to Degrees1/1
  Radians to Degrees/1 -> Wind and Turbulence/3(lonx)
  Radians to Degrees1/1 -> Wind and Turbulence/2(latx)
  lon/1 -> Radians to Degrees/1
  Wind and Turbulence/2(VBAB) -> VBAB/1
  Square/1 -> Product/2
  Product/1 -> Gain/1
  Gain/1 -> pdynmc/1
  TBD/1 -> Wind and Turbulence/5(TBD)
  alppx/1 -> Wind and Turbulence/6(alppx)
  phipx/1 -> Wind and Turbulence/7(phipx)

== system GHAME_Model_2018b/GHAME Airframe/Forces and Moments/AERODYNAMICS ==
  Deflections : Inport
  Mach number : Inport  Port=2
  Airspeed : Inport  Port=3
  Angle of attack : Inport  Port=4
  Sideslip angle : Inport  Port=5
  Angular velocity : Inport  Port=6
  Aerodynamic Coefficients : MATLAB Function  TreatAsAtomicUnit=on
  Bus Creator2 : BusCreator  Inputs=4
  Aero: Data : Outport
  wires:
  Mach number/1 -> Aerodynamic Coefficients/2(vmach)
  Aerodynamic Coefficients/2(c_moment) -> Bus Creator2/2  "Moment coefficients"
  Airspeed/1 -> Aerodynamic Coefficients/3(DVBA)
  Aerodynamic Coefficients/4(cxz) -> Bus Creator2/4  "Aero: force coefficients"
  Angle of attack/1 -> Aerodynamic Coefficients/4(alphax)
  Aerodynamic Coefficients/1(c_force) -> Bus Creator2/1  "Force coefficients"
  Aerodynamic Coefficients/3(cmu) -> Bus Creator2/3  "Control derivatives"
  Deflections/1 -> Aerodynamic Coefficients/1(delta)
  Bus Creator2/1 -> Aero: Data/1
  Angular velocity/1 -> Aerodynamic Coefficients/6(WBEBx)
  Sideslip angle/1 -> Aerodynamic Coefficients/5(betax)

== system GHAME_Model_2018b/GHAME Airframe/Forces and Moments/FORCE ==
  Prop: data : Inport
  Aero: Data : Inport  Port=2
  Aerodynamic moments : MATLAB Function  TreatAsAtomicUnit=on
  Bus Selector : BusSelector  OutputSignals=Thrust,Dynamic pressure
  Bus Selector1 : BusSelector  OutputSignals=Force coefficients,Moment coefficients
  Non-gravitational forces : MATLAB Function  TreatAsAtomicUnit=on
  FMB : Outport
  FAPB : Outport  Port=2
  wires:
  Prop: data/1 -> Bus Selector/1
  Bus Selector/2 -> Non-gravitational forces/2(pdynmc), Aerodynamic moments/2(pdynmc)  "<Dynamic pressure>"
  Non-gravitational forces/1(FAPB) -> FAPB/1
  Bus Selector1/1 -> Non-gravitational forces/3(c_force)  "<Force coefficients>"
  Aerodynamic moments/1(FMB) -> FMB/1
  Bus Selector/1 -> Non-gravitational forces/1(Thrust)  "<Thrust>"
  Aero: Data/1 -> Bus Selector1/1
  Bus Selector1/2 -> Aerodynamic moments/1(c_moment)  "<Moment coefficients>"

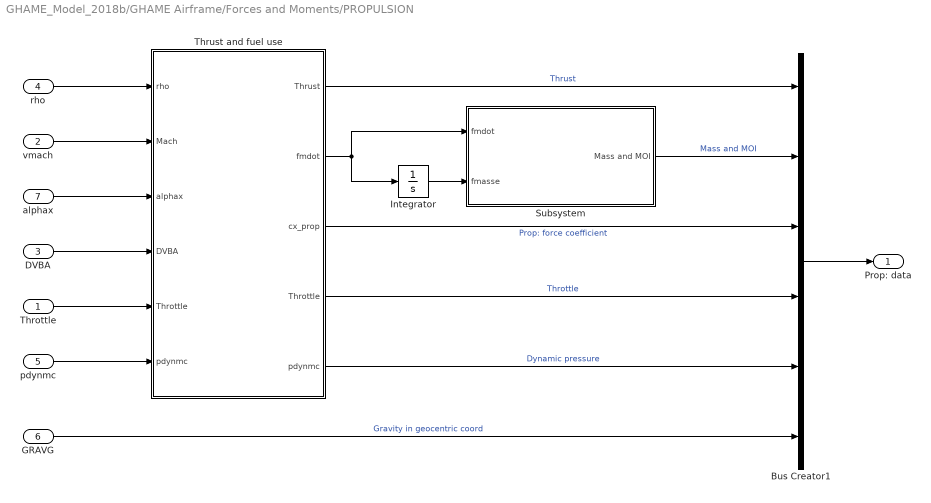
== system GHAME_Model_2018b/GHAME Airframe/Forces and Moments/PROPULSION ==
  Throttle : Inport
  vmach : Inport  Port=2
  DVBA : Inport  Port=3
  rho : Inport  Port=4
  pdynmc : Inport  Port=5
  GRAVG : Inport  Port=6
  alphax : Inport  Port=7
  Bus Creator1 : BusCreator  Inputs=6
  Integrator : Integrator
  Subsystem : Subsystem
  Thrust and fuel use : MATLAB Function  TreatAsAtomicUnit=on
  Prop: data : Outport
  wires:
  alphax/1 -> Thrust and fuel use/3(alphax)
  Thrust and fuel use/2(fmdot) -> Integrator/1, Subsystem/1(fmdot)
  pdynmc/1 -> Thrust and fuel use/6("pdynmc ")
  vmach/1 -> Thrust and fuel use/2(Mach)
  rho/1 -> Thrust and fuel use/1(rho)
  DVBA/1 -> Thrust and fuel use/4(DVBA)
  Thrust and fuel use/3(cx_prop) -> Bus Creator1/3  "Prop: force coefficient"
  Thrust and fuel use/1(Thrust) -> Bus Creator1/1  "Thrust"
  Throttle/1 -> Thrust and fuel use/5("Throttle ")
  Bus Creator1/1 -> Prop: data/1
  Thrust and fuel use/4(Throttle) -> Bus Creator1/4  "Throttle"
  Thrust and fuel use/5(pdynmc) -> Bus Creator1/5  "Dynamic pressure"
  GRAVG/1 -> Bus Creator1/6  "Gravity in geocentric coord"
  Integrator/1 -> Subsystem/2(fmasse)
  Subsystem/1(Mass and MOI) -> Bus Creator1/2  "Mass and MOI"

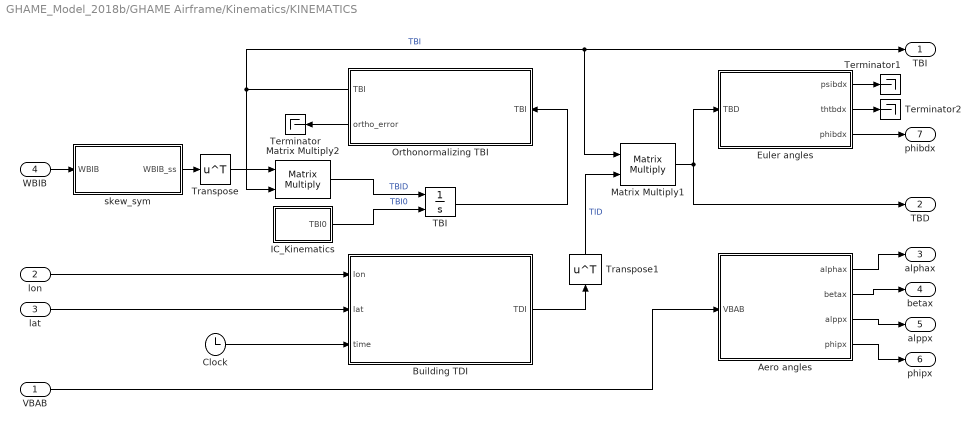
== system GHAME_Model_2018b/GHAME Airframe/Kinematics/KINEMATICS ==
  VBAB : Inport
  lon : Inport  Port=2
  lat : Inport  Port=3
  WBIB : Inport  Port=4
  "\tOrthonormalizing TBI " : MATLAB Function  TreatAsAtomicUnit=on
  Aero angles : MATLAB Function  TreatAsAtomicUnit=on
  Building TDI : MATLAB Function  TreatAsAtomicUnit=on
  Clock : Clock
  Euler angles : MATLAB Function  TreatAsAtomicUnit=on
  IC_Kinematics : Subsystem
  Matrix Multiply1 : Product  Multiplication=Matrix(*)
  Matrix Multiply2 : Product  Multiplication=Matrix(*)
  "TBI  " : Integrator  InitialConditionSource=external  InitialCondition=v0_BE_B
  Terminator : Terminator
  Terminator1 : Terminator
  Terminator2 : Terminator
  Transpose : Math  Operator=transpose  SaturateOnIntegerOverflow=on
  Transpose1 : Math  Operator=transpose  SaturateOnIntegerOverflow=on
  skew_sym : MATLAB Function  TreatAsAtomicUnit=on
  "TBI " : Outport
  TBD : Outport  Port=2
  alphax : Outport  Port=3
  betax : Outport  Port=4
  alppx : Outport  Port=5
  phipx : Outport  Port=6
  phibdx : Outport  Port=7
  wires:
  Clock/1 -> Building TDI/3(time)
  WBIB/1 -> skew_sym/1(WBIB)
  Euler angles/2(thtbdx) -> Terminator2/1
  lat/1 -> Building TDI/2(lat)
  Building TDI/1(TDI) -> Transpose1/1
  Euler angles/3(phibdx) -> phibdx/1
  "\tOrthonormalizing TBI "/1(TBI) -> Matrix Multiply2/2, "TBI "/1, Matrix Multiply1/1  "TBI"
  Matrix Multiply1/1 -> Euler angles/1(TBD), TBD/1
  skew_sym/1(WBIB_ss) -> Transpose/1
  lon/1 -> Building TDI/1(lon)
  "\tOrthonormalizing TBI "/2(ortho_error) -> Terminator/1
  Transpose1/1 -> Matrix Multiply1/2  "TID"
  Euler angles/1(psibdx) -> Terminator1/1
  Transpose/1 -> Matrix Multiply2/1
  Matrix Multiply2/1 -> "TBI  "/1  "TBID"
  IC_Kinematics/1(TBI0) -> "TBI  "/2  "TBI0"
  "TBI  "/1 -> "\tOrthonormalizing TBI "/1("TBI ")
  VBAB/1 -> Aero angles/1(VBAB)
  Aero angles/1(alphax) -> alphax/1
  Aero angles/2(betax) -> betax/1
  Aero angles/3(alppx) -> alppx/1
  Aero angles/4(phipx) -> phipx/1

== system GHAME_Model_2018b/GHAME Airframe/Dynamics/EULER/Cross product ==
  A : Inport
  B : Inport  Port=2
  Subsystem : sharedutil/3x3 Cross Product/Subsystem  SystemSampleTime=-1  Latency=0  AutoFrameSizeCalculation=off
  Subsystem1 : sharedutil/3x3 Cross Product/Subsystem1  SystemSampleTime=-1  Latency=0  AutoFrameSizeCalculation=off
  Sum : Sum  Inputs=+|-  InputSameDT=on  SaturateOnIntegerOverflow=on  OutDataTypeStr=Inherit: Same as first input
  Out1 : Outport
  wires:
  A/1 -> Subsystem1/1, Subsystem/1
  B/1 -> Subsystem1/2, Subsystem/2
  Subsystem1/1 -> Sum/2
  Sum/1 -> Out1/1
  Subsystem/1 -> Sum/1

== system GHAME_Model_2018b/GHAME Airframe/Dynamics/EULER/Initial body rate ==
  Constant : Constant  Value=IC.WBIB
  WBIB0 : Outport
  wires:
  Constant/1 -> WBIB0/1

== system GHAME_Model_2018b/GHAME Airframe/Dynamics/NEWTON/Geodetic position update ==
  SBII : Inport
  Clock : Clock
  Geodetic Position : MATLAB Function  TreatAsAtomicUnit=on
  TM Inertial to Geocentric : MATLAB Function  TreatAsAtomicUnit=on
  TM Inertial to Geodetic : MATLAB Function  TreatAsAtomicUnit=on
  TGI : Outport
  TDI : Outport  Port=2
  lon : Outport  Port=3
  lat : Outport  Port=4
  alt : Outport  Port=5
  wires:
  SBII/1 -> Geodetic Position/2(SBII)
  Geodetic Position/1(lon) -> lon/1
  Geodetic Position/3(lat) -> TM Inertial to Geodetic/2("lat ")
  TM Inertial to Geodetic/1(TDI) -> TM Inertial to Geocentric/1("TDI ")
  Clock/1 -> Geodetic Position/1(time)
  TM Inertial to Geocentric/1(TGI) -> TGI/1
  Geodetic Position/2(lon_cel) -> TM Inertial to Geodetic/1(lon_cel)
  TM Inertial to Geocentric/4(alt) -> alt/1
  TM Inertial to Geocentric/3(lat) -> lat/1
  TM Inertial to Geocentric/2(TDI) -> TDI/1
  TM Inertial to Geodetic/2(lat) -> TM Inertial to Geocentric/2("lat ")
  Geodetic Position/4(alt) -> TM Inertial to Geocentric/3("alt ")

== system GHAME_Model_2018b/GHAME Airframe/Dynamics/NEWTON/Initial inertial pos. ==
  Constant : Constant  Value=IC.SBII
  SBII0 : Outport
  wires:
  Constant/1 -> SBII0/1

== system GHAME_Model_2018b/GHAME Airframe/Dynamics/NEWTON/Initial inertial vel. ==
  Constant : Constant  Value=IC.VBII
  VBII0 : Outport
  wires:
  Constant/1 -> VBII0/1

== system GHAME_Model_2018b/GHAME Airframe/Dynamics/NEWTON/Speed ==
  VBED [NED] : Inport
  Dot Product : DotProduct  InputSameDT=on  OutDataTypeStr=Inherit: Inherit via internal rule
  Square Root : Sqrt  SaturateOnIntegerOverflow=on
  DVBE : Outport
  wires:
  VBED [NED]/1 -> Dot Product/2, Dot Product/1
  Dot Product/1 -> Square Root/1
  Square Root/1 -> DVBE/1

== system GHAME_Model_2018b/GHAME Airframe/Environment/ENVIRONMENT/Stop Simulation when alt < 0 ==
  alt : Inport
  If : If  IfExpression=u1 <= 25  ShowElse=off
  Stop Simulationalt<0 : Subsystem  TreatAsAtomicUnit=on
  wires:
  If/1 -> Stop Simulationalt<0/Action
  alt/1 -> If/1

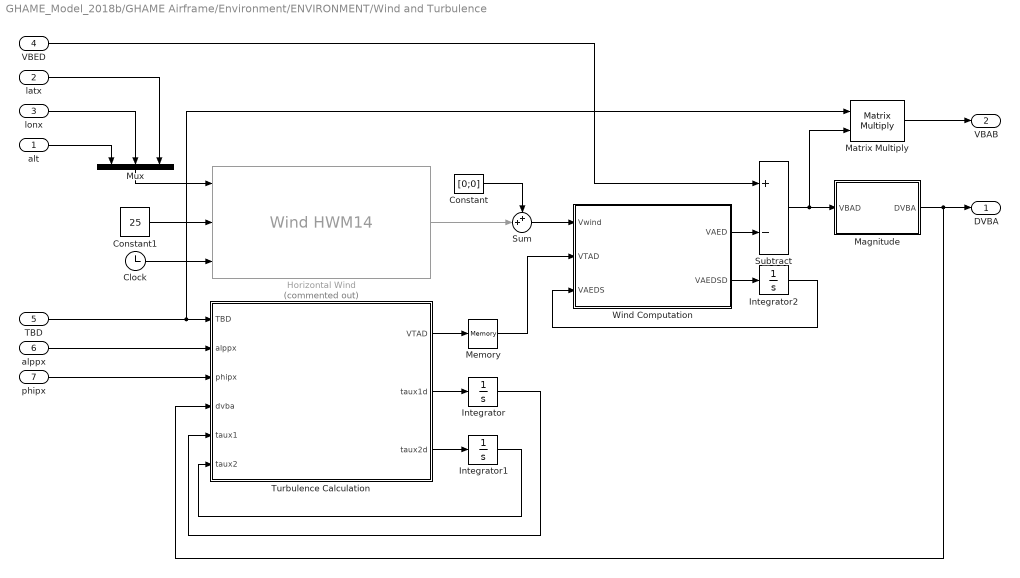
== system GHAME_Model_2018b/GHAME Airframe/Environment/ENVIRONMENT/Wind and Turbulence ==
  alt : Inport
  latx : Inport  Port=2
  lonx : Inport  Port=3
  VBED : Inport  Port=4
  TBD : Inport  Port=5
  alppx : Inport  Port=6
  phipx : Inport  Port=7
  Clock : Clock
  Constant : Constant  Value=[0;0]
  Constant1 : Constant  Value=25
  Horizontal Wind : WindHWM14  Commented=on
  Integrator : Integrator
  Integrator1 : Integrator
  Integrator2 : Integrator  InitialCondition=[0; 0; 0]
  Magnitude : MATLAB Function  TreatAsAtomicUnit=on
  Matrix Multiply : Product  Multiplication=Matrix(*)
  Memory : Memory  InitialCondition=[0; 0; 0]
  Mux : Mux  Inputs=3
  Subtract : Sum  Inputs=+-
  Sum : Sum  Inputs=++|
  Turbulence Calculation : MATLAB Function  TreatAsAtomicUnit=on
  Wind Computation : MATLAB Function  TreatAsAtomicUnit=on
  DVBA : Outport
  VBAB : Outport  Port=2
  wires:
  alt/1 -> Mux/1
  lonx/1 -> Mux/2
  Mux/1 -> Horizontal Wind/1
  Turbulence Calculation/2(taux1d) -> Integrator/1
  alppx/1 -> Turbulence Calculation/2(alppx)
  TBD/1 -> Turbulence Calculation/1(TBD), Matrix Multiply/1
  Clock/1 -> Horizontal Wind/3
  phipx/1 -> Turbulence Calculation/3(phipx)
  Constant1/1 -> Horizontal Wind/2
  Integrator2/1 -> Wind Computation/3(VAEDS)
  Subtract/1 -> Magnitude/1(VBAD), Matrix Multiply/2
  Integrator1/1 -> Turbulence Calculation/6(taux2)
  Integrator/1 -> Turbulence Calculation/5(taux1)
  Turbulence Calculation/3(taux2d) -> Integrator1/1
  latx/1 -> Mux/3
  VBED/1 -> Subtract/1
  Wind Computation/1(VAED) -> Subtract/2
  Wind Computation/2(VAEDSD) -> Integrator2/1
  Magnitude/1(DVBA) -> DVBA/1, Turbulence Calculation/4(dvba)
  Matrix Multiply/1 -> VBAB/1
  Turbulence Calculation/1(VTAD) -> Memory/1
  Horizontal Wind/1 -> Sum/2
  Memory/1 -> Wind Computation/2(VTAD)
  Sum/1 -> Wind Computation/1(Vwind)
  Constant/1 -> Sum/1

== system GHAME_Model_2018b/GHAME Airframe/Forces and Moments/PROPULSION/Subsystem ==
  fmdot : Inport
  fmasse : Inport  Port=2
  Bus Creator : BusCreator  Inputs=3
  Stop Simulation : Stop
  Updating mass and inertia : MATLAB Function  TreatAsAtomicUnit=on
  Mass and MOI : Outport
  wires:
  Updating mass and inertia/3(vmass) -> Bus Creator/3  "Vehicle mass"
  Updating mass and inertia/4(stop_flag) -> Stop Simulation/1
  fmasse/1 -> Updating mass and inertia/2(fmasse)
  Updating mass and inertia/2(IBBBdot) -> Bus Creator/2  "MOI derivative"
  fmdot/1 -> Updating mass and inertia/1(fmdot)
  Updating mass and inertia/1(IBBB) -> Bus Creator/1  "MOI"
  Bus Creator/1 -> Mass and MOI/1

== system GHAME_Model_2018b/GHAME Airframe/Kinematics/KINEMATICS/IC_Kinematics ==
  Constant : Constant  Value=IC.TBI
  TBI0 : Outport
  wires:
  Constant/1 -> TBI0/1

== system GHAME_Model_2018b/GHAME Airframe/Environment/ENVIRONMENT/Stop Simulation when alt < 0/Stop Simulationalt<0 ==
  Action Port : ActionPort
  Constant2 : Constant
  Stop Simulation : Stop
  wires:
  Constant2/1 -> Stop Simulation/1

== matlab function GHAME_Model_2018b/GHAME Airframe/Forces and Moments/AERODYNAMICS/Aerodynamic Coefficients ==
  data: delta input; vmach input; DVBA input; c_force output double size=[3 1]; alphax input; betax input; WBEBx input; c_moment output double size=[3 1]; Data parameter; Sim parameter; UNC parameter; cmu output; cxz output
function [c_force, c_moment, cmu, cxz] = aerodynamics(delta, vmach, DVBA, alphax, betax, WBEBx, Data, Sim, UNC)
                                                       
% Conversions
RAD = Sim.constants.RAD;
DEG = Sim.constants.DEG;

refb = Sim.vehicle.geometry.refb;
refc = Sim.vehicle.geometry.refc;

delax = delta(1)*DEG;
delex = delta(2)*DEG;
delrx = delta(3)*DEG;

ppx = WBEBx(1);
qqx = WBEBx(2);
rrx = WBEBx(3);

% Breakpoints
alpha_vec    = (-3:3:+21);
mach_vec     = [0.4 0.6 0.8 0.9 0.95 1.05 1.2 1.5 2.0 3.0 6.0 12.0 24.0];

% Helper function for interpolation
interp_coeff = @(table) interp2(mach_vec, alpha_vec, table, ...
    clamp_value(vmach, mach_vec(1), mach_vec(end)), ...
    clamp_value(alphax, alpha_vec(1), alpha_vec(end)), ...
    'linear');

if Sim.mode.muncertainty == 1
    % Uncertainty enabled → use perturbed coefficients
    AeroData     = UNC.Perturbed;
    AeroData_Nom = UNC.Nominal;
else
    % Uncertainty disabled → use nominal coefficients
    AeroData     = Data.AeroCoefficients;
    AeroData_Nom = Data.AeroCoefficients;
end

% Coefficients
CL1_tab     =   AeroData.CL1_tab;
Cm1_tab     =   AeroData.Cm1_tab;
CD1_tab     =   AeroData.CD1_tab;

%%% Interpolated aerodynamic coefficients %%%

% Indexed model
Cm1 = interp2(mach_vec, alpha_vec, Cm1_tab,  vmach, alphax, 'linear');
CL1 = interp2(mach_vec, alpha_vec, CL1_tab,  vmach, alphax, 'linear');
CD1 = interp2(mach_vec, alpha_vec, CD1_tab,  vmach, alphax, 'linear');

% Drag
cd0 = interp_coeff(AeroData.CD0_tab);
cda = interp_coeff(AeroData.CDA_tab);
cd  = CD1 ;

% Lift
cl0  = interp_coeff(AeroData.CL0_tab);
cla  = interp_coeff(AeroData.CLA_tab);
clde = interp_coeff(AeroData.CLDE_tab);
cl   = (CL1 + clde * delex);

% Side force
cyb  = interp_coeff(AeroData.CYB_tab);
cyda = interp_coeff(AeroData.CYDA_tab);
cydr = interp_coeff(AeroData.CYDR_tab);
cy   = cyb * betax + cyda * delax + cydr * delrx;

% Rolling moment
cllb  = interp_coeff(AeroData.CLLB_tab)  ;
cllda = interp_coeff(AeroData.CLLDA_tab);
clldr = interp_coeff(AeroData.CLLDR_tab);
cllp  = interp_coeff(AeroData.CLLP_tab);
cllr  = interp_coeff(AeroData.CLLR_tab);
cll   = cllb * betax + cllda * delax + clldr * delrx + ...
        cllp * ppx * RAD * refb / (2 * DVBA) + cllr * rrx * RAD * refb / (2 * DVBA);

% Pitching moment
cm0   = interp_coeff(AeroData.CM0_tab);
cma   = interp_coeff(AeroData.CMA_tab);
cmde  = interp_coeff(AeroData.CMDE_tab) ;
cmq   = interp_coeff(AeroData.CMQ_tab)  ;
clm   = Cm1 + cmde * delex + cmq * qqx * RAD * refc / (2 * DVBA);

% Yawing moment
clnb  = interp_coeff(AeroData.CNB_tab) ;
clnda = interp_coeff(AeroData.CNDA_tab);
clndr = interp_coeff(AeroData.CNDR_tab);
clnp  = interp_coeff(AeroData.CNP_tab) ;
clnr  = interp_coeff(AeroData.CNR_tab) ;
cln   = clnb * betax + clnda * delax + clndr * delrx + ...
        clnp * ppx * RAD * refb / (2 * DVBA) + clnr * rrx * RAD * refb / (2 * DVBA);

% Force coefficients in body coords
cosa = cos(alphax*RAD);
sina = sin(alphax*RAD);

cx = -cd * cosa + cl * sina;
cz = -cd * sina - cl * cosa;

c_force  = [cx; cy; cz];
c_moment = [cll; clm; cln];

%%% ====================================================================
%%% CONTROLLER-RELATED TERMS (always nominal, no uncertainty)
%%% ====================================================================

cmde_nom = interp_coeff(AeroData_Nom.CMDE_tab);
cda_nom  = interp_coeff(AeroData_Nom.CDA_tab);
cla_nom  = interp_coeff(AeroData_Nom.CLA_tab);

cmu = [refb*interp_coeff(AeroData_Nom.CLLDA_tab), 0, refb*interp_coeff(AeroData_Nom.CLLDR_tab);
       0, refc * cmde_nom, 0;
       refb*interp_coeff(AeroData_Nom.CNDA_tab), 0, refb*interp_coeff(AeroData_Nom.CNDR_tab)];

cxa = -cda_nom * cosa + cla_nom * sina;
cza = -cda_nom * sina - cla_nom * cosa;

cxz = [cxa; cza];

end

%% Helper function
function value_clamped = clamp_value(value, min_value, max_value)
    value_clamped = max(min(value, max_value), min_value);
end

== matlab function GHAME_Model_2018b/GHAME Airframe/Environment/ENVIRONMENT/Wind and Turbulence/Magnitude ==
  data: VBAD input; DVBA output
function DVBA = fcn(VBAD)
% Calculates magnitude of vector

DVBA = sqrt(VBAD(1)^2+VBAD(2)^2+VBAD(3)^2);

== matlab function GHAME_Model_2018b/GHAME Airframe/Forces and Moments/FORCE/Non-gravitational forces ==
  data: Thrust input; pdynmc input; c_force input; FAPB output size=[3 1]; Sim parameter
function FAPB = computeForces(Thrust, pdynmc, c_force, Sim)
% computeForces
% -------------------------------------------------------------------------
% Computes the total non-gravitational forces acting on the vehicle in the
% body coordinate system. These include the aerodynamic force components
% and the propulsive contribution along the body x-axis.
%
% INPUTS:
%   thrust  - Propulsive thrust force along body x-axis [N]
%   pdynmc  - Dynamic pressure [Pa]

    refa = Sim.vehicle.geometry.refa;
    cx = c_force(1);
    cy = c_force(2);
    cz = c_force(3);
%
% OUTPUT:
%   FAPB    - 3x1 vector of total non-gravitational forces in the body
%             coordinate system [N]
%             FAPB = [F_x; F_y; F_z]
%

    FAPB = [pdynmc * refa * cx + Thrust;   % Body x-force (aero + thrust)
            pdynmc * refa * cy;            % Body y-force (aero only)
            pdynmc * refa * cz];           % Body z-force (aero only)
end

== matlab function GHAME_Model_2018b/GHAME Airframe/Environment/ENVIRONMENT/Wind and Turbulence/Turbulence Calculation ==
  settings: updateMethod=DISCRETE
  data: TBD input; alppx input; phipx input; dvba input; taux1 input; taux2 input; VTAD output; taux1d output; taux2d output; Sim parameter
function [VTAD, taux1d, taux2d] = environment_dryden(TBD, alppx, phipx, dvba, taux1, taux2, Sim)
    % ENVIRONMENT_DRYDEN Simulates Dryden turbulence in geodetic coordinates.
    %
    % Inputs:
    %   dvba      - Airspeed magnitude [scalar]
    %   Ts  - Integration step size [scalar]
    %   round6    - Data storage (provides turbulence parameters)
    %   taux1, taux1d, taux2, taux2d - Turbulence state variables
    %
    % Outputs:
    %   VTAD - Turbulence velocity in geodetic coordinates [3x1]
    %   taux1_new, taux1d_new, taux2_new, taux2d_new - Updated turbulence states

    % Constants
    PI  = Sim.constants.PI;
    RAD = Sim.constants.RAD;

    Ts = Sim.sample_time;
    
    turb_sigma  = Sim.wind.turb_sigma; 
    turb_length = Sim.wind.turb_length;

    % Generate white Gaussian noise with zero mean
    value1 = 0;
    while value1 == 0
        value1 = rand;
    end
    value2 = rand;
    gauss_value = (1 / sqrt(Ts)) * sqrt(2 * log(1 / value1)) * cos(2 * PI * value2);

    % Dryden turbulence filtering
    vl = dvba / turb_length;

    % Integrate first state variable
    taux1d = taux2;
    
    % Integrate second state variable
    taux2d = -vl^2 * taux1 - 2 * vl * taux2 + vl^2 * gauss_value;

    % Compute turbulence variable `tau`
    tau = turb_sigma * sqrt(1 / (vl * PI)) * (taux1 + sqrt(3) * taux2 / vl);

    % Transform turbulence to body coordinates
    VTAB = [-tau * sin(alppx * RAD);
             tau * sin(phipx * RAD) * cos(alppx * RAD);
             tau * cos(phipx * RAD) * cos(alppx * RAD)];

    % Convert to geodetic coordinates
    VTAD = TBD * VTAB;
end
